simulink model "sersin"  (R2015a)
settings: Solver=FixedStepDiscrete  StartTime=0.0  StopTime=100  FixedStep=0.01  RelTol=1e-3
libraries: simulink x3, arduinolib x3
settings Model: ExtModeTrigDuration=2  Creator=pela  LastModifiedBy=pela
settings OptimizationCC: OptimizeModelRefInitCode=on  LifeSpan=1
settings DebuggingCC: UnderspecifiedInitializationDetection=Classic  MergeDetectMultiDrivingBlocksExec=none
settings HardwareCC: ProdBitPerInt=16  ProdBitPerPointer=8  ProdIntDivRoundTo=Zero  ProdEndianess=LittleEndian  ProdWordSize=8  ProdHWDeviceType=Atmel->AVR
settings RTWCC: SystemTargetFile=realtime.tlc  GenerateMakefile=off  TemplateMakefile=realtime.tmf  Description=Run on Target Hardware  RTWVerbose=off
settings ERTTargetCC: CombineOutputUpdateFcns=off  ExtModeTransport=3  ExtModeMexFile=ext_serial_win32_comm_rtt  ExtModeMexArgs=0 1 9600  ERTSrcFileBannerTemplate=realtime_code_template.cgt  ERTHdrFileBannerTemplate=realtime_code_template.cgt  ERTDataSrcFileTemplate=realtime_code_template.cgt  ERTDataHdrFileTemplate=realtime_code_template.cgt  ERTCustomFileTemplate=realtime_file_process.tlc

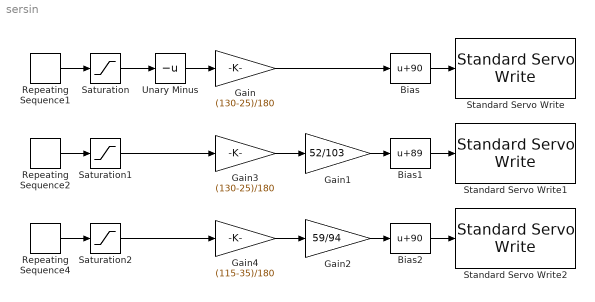
== system sersin ==
  Bias : Bias  Bias=90
  Bias1 : Bias  Bias=89
  Bias2 : Bias  Bias=90
  Gain : Gain  Gain=(130-25)/180
  Gain1 : Gain  Gain=52/103
  Gain2 : Gain  Gain=59/94
  Gain3 : Gain  Gain=(130-25)/180
  Gain4 : Gain  Gain=(115-35)/180
  Repeating Sequence1 : simulink/Sources/Repeating Sequence  rep_seq_t=[0 1 2 3 4 5 6 7 8 9 10 11 12 13 14 15 16]  rep_seq_y=[-90 -90 -45 -45 0 0 45 45 90 90 45 45 0 0 -45 -45 -90]
  Repeating Sequence2 : simulink/Sources/Repeating Sequence  rep_seq_t=[0 7 8 (2*8-1) (2*8) (3*8-1) (3*8) (4*8-1) (4*8) (5*8-1) (5*8) (6*8-1) (6*8) (7*8-1) (7*8) (8*8-1) (8*8) (9*8-1) (9*8) (10*8-1) (10*8) (11*8-1) (11*8) (12*8-1) (12*8) (13*8-1) (13*8) (14*8-1) (14*8) (15*8-1) (15*8) (16*8-1) (16*8)]  rep_seq_y=[0 0 45 45 90 90 135 135 180 180 135 135 90 90 45 45 0 0 -45 -45 -90 -90 -135 -135 -180 -180 -135 -135 -90 -90 -45 -45 0]
  Repeating Sequence4 : simulink/Sources/Repeating Sequence  rep_seq_t=[0 128-1 128 (2*128-1) (2*128+1) (3*128-1) (3*128+1) (4*128-1) (4*128+1) (5*128-1)]  rep_seq_y=[180 180 90 90 0 0 -90 -90 -180 -180]
  Saturation : Saturate  UpperLimit=90  LowerLimit=-90
  Saturation1 : Saturate  UpperLimit=180  LowerLimit=-180
  Saturation2 : Saturate  UpperLimit=180  LowerLimit=-180
  Standard Servo Write : arduinolib/Standard Servo Write  pinNumber=9  blockPlatform=arduino
  Standard Servo Write1 : arduinolib/Standard Servo Write  pinNumber=10  blockPlatform=arduino
  Standard Servo Write2 : arduinolib/Standard Servo Write  pinNumber=11  blockPlatform=arduino
  Unary Minus : UnaryMinus
  wires:
  Repeating Sequence4/1 -> Saturation2/1
  Gain1/1 -> Bias1/1
  Gain2/1 -> Bias2/1
  Saturation/1 -> Unary Minus/1
  Gain/1 -> Bias/1
  Bias1/1 -> Standard Servo Write1/1
  Bias/1 -> Standard Servo Write/1
  Bias2/1 -> Standard Servo Write2/1
  Gain3/1 -> Gain1/1
  Gain4/1 -> Gain2/1
  Repeating Sequence2/1 -> Saturation1/1
  Repeating Sequence1/1 -> Saturation/1
  Unary Minus/1 -> Gain/1
  Saturation1/1 -> Gain3/1
  Saturation2/1 -> Gain4/1
